simulink model "Suspension2_26_09_2023"  (R2022a)
settings: Solver=FixedStepAuto  StartTime=0.0  StopTime=10.0  FixedStep=0.001  RelTol=1e-3
undefined symbols (not defined in the file): a, alpha, area, b, beta, c, Force_rear_tyre, gamma, k, m, niu, theta1, theta2
libraries: simulink x1
settings Model: Creator=oltea  LastModifiedBy=oltea
settings DataIOCC: ReturnWorkspaceOutputs=off

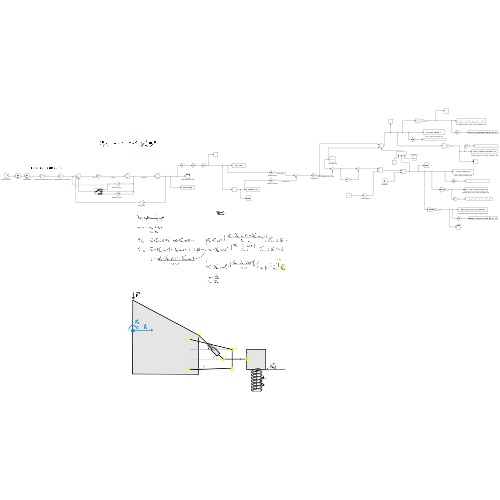
[thumbnail: Simulink's stored preview of the top-level diagram]
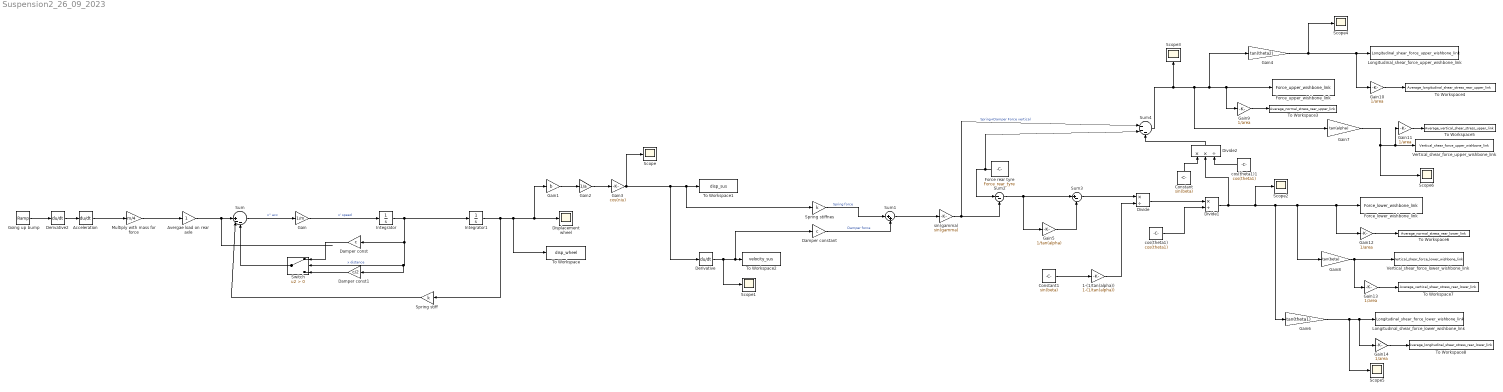
== system Suspension2_26_09_2023 ==
  " Avergae load on rear axle" : Gain
  1-(1/tan(alpha)) : Gain  Gain=1-(1/tan(alpha))
  Acceleration : Derivative
  Constant : Constant  Value=sin(beta)
  Constant1 : Constant  Value=sin(beta)
  Damper const : Gain  Gain=c
  Damper const1 : Gain  Gain=c/2
  Damper constant : Gain  Gain=c
  Derivative : Derivative
  Derivative2 : Derivative
  Displacement wheel : Scope
  Divide : Product  Inputs=*/
  Divide1 : Product  Inputs=*/
  Divide2 : Product  Inputs=**/
  Force rear tyre : Constant  Value=Force_rear_tyre
  Force_lower_wishbone_link : ToWorkspace  VariableName=Force_lower_wishbone_link  SampleTime=-1
  Force_upper_wishbone_link : ToWorkspace  VariableName=Force_upper_wishbone_link  SampleTime=-1
  Gain : Gain  Gain=1/m
  Gain1 : Gain  Gain=b
  Gain{9..14} (6 alike) : Gain  Gain=1/area
  Gain2 : Gain  Gain=1/a
  Gain3 : Gain  Gain=cos(niu)
  Gain4 : Gain  Gain=tan(theta2)
  Gain5 : Gain  Gain=1/tan(alpha)
  Gain6 : Gain  Gain=tan(theta1)
  Gain7 : Gain  Gain=tan(alpha)
  Gain8 : Gain  Gain=tan(beta)
  Going up bump : simulink/Sources/Ramp  slope=0.42  start=0  InitialOutput=7
  Integrator : Integrator
  Integrator1 : Integrator
  Longitudinal_shear_force_lower_wishbone_link : ToWorkspace  VariableName=Longitudinal_shear_force_lower_wishbone_link  SampleTime=-1
  Longitudinal_shear_force_upper_wishbone_link : ToWorkspace  VariableName=Longitudinal_shear_force_upper_wishbone_link  SampleTime=-1
  Multiply with mass for force : Gain  Gain=m/4
  Scope{,1..6} (7 alike) : Scope
  Spring stiff : Gain  Gain=k
  Spring stiffnes : Gain  Gain=k
  Sum : Sum  Inputs=||+--
  Sum1 : Sum  Inputs=|++
  Sum2 : Sum  Inputs=|--
  Sum3 : Sum  Inputs=|+-
  Sum4 : Sum  Inputs=|---
  Switch : Switch  Criteria=u2 > Threshold  SaturateOnIntegerOverflow=off  InputSameDT=off
  To Workspace : ToWorkspace  VariableName=disp_wheel  SampleTime=-1
  To Workspace1 : ToWorkspace  VariableName=disp_sus  SampleTime=-1
  To Workspace2 : ToWorkspace  VariableName=velocity_sus  SampleTime=-1
  To Workspace3 : ToWorkspace  VariableName=Average_normal_stress_rear_upper_link  SampleTime=-1
  To Workspace4 : ToWorkspace  VariableName=Average_longitudinal_shear_stress_rear_upper_link  SampleTime=-1
  To Workspace5 : ToWorkspace  VariableName=Average_vertical_shear_stress_upper_link  SampleTime=-1
  To Workspace6 : ToWorkspace  VariableName=Average_normal_stress_rear_lower_link  SampleTime=-1
  To Workspace7 : ToWorkspace  VariableName=Average_vertical_shear_stress_rear_lower_link  SampleTime=-1
  To Workspace8 : ToWorkspace  VariableName=Average_longitudinal_shear_stress_rear_lower_link  SampleTime=-1
  Vertical_shear_force_lower_wishbone_link : ToWorkspace  VariableName=Vertical_shear_force_lower_wishbone_link  SampleTime=-1
  Vertical_shear_force_upper_wishbone_link : ToWorkspace  VariableName=Vertical_shear_force_upper_wishbone_link  SampleTime=-1
  cos(theta1) : Constant  Value=cos(theta1)
  cos(theta1)1 : Constant  Value=cos(theta1)
  sin(gamma) : Gain  Gain=sin(gamma)
  wires:
  Switch/1 -> Sum/3
  Damper const1/1 -> Switch/3
  Spring stiff/1 -> Sum/2
  Integrator/1 -> Damper const1/1, Switch/2, Damper const/1, Integrator1/1  "x distance"
  Integrator1/1 -> Spring stiff/1, To Workspace/1, Gain1/1, Displacement wheel/1
  Damper const/1 -> Switch/1
  Sum/1 -> Gain/1  "x'' acc"
  Gain/1 -> Integrator/1  "x' speed"
  Going up bump/1 -> Derivative2/1
  Derivative2/1 -> Acceleration/1
  Acceleration/1 -> Multiply with mass for force/1
  Gain1/1 -> Gain2/1
  Gain2/1 -> Gain3/1
  Gain3/1 -> Scope/1, Derivative/1, Spring stiffnes/1, To Workspace1/1
  Derivative/1 -> Scope1/1, Damper constant/1, To Workspace2/1
  Spring stiffnes/1 -> Sum1/1  "Spring force"
  Damper constant/1 -> Sum1/2  "Damper force"
  Sum1/1 -> sin(gamma)/1
  Force rear tyre/1 -> Sum4/2, Sum2/1
  sin(gamma)/1 -> Sum4/1, Sum2/2  "Spring+Damper Force vertical"
  Sum2/1 -> Gain5/1, Sum3/1
  Gain5/1 -> Sum3/2
  Sum3/1 -> Divide/1
  1-(1/tan(alpha))/1 -> Divide/2
  Divide/1 -> Divide1/1
  cos(theta1)/1 -> Divide1/2
  Divide1/1 -> Scope2/1, Gain6/1, Gain8/1, Gain12/1, Force_lower_wishbone_link/1, Divide2/2
  Constant1/1 -> 1-(1/tan(alpha))/1
  Sum4/1 -> Gain7/1, Gain4/1, Gain9/1, Force_upper_wishbone_link/1, Scope3/1
  Constant/1 -> Divide2/1
  Divide2/1 -> Sum4/3
  cos(theta1)1/1 -> Divide2/3
  Gain4/1 -> Scope4/1, Gain10/1, Longitudinal_shear_force_upper_wishbone_link/1
  Gain6/1 -> Scope5/1, Gain14/1, Longitudinal_shear_force_lower_wishbone_link/1
  Gain7/1 -> Scope6/1, Gain11/1, Vertical_shear_force_upper_wishbone_link/1
  Gain8/1 -> Gain13/1, Vertical_shear_force_lower_wishbone_link/1
  Gain9/1 -> To Workspace3/1
  Gain10/1 -> To Workspace4/1
  Gain11/1 -> To Workspace5/1
  Gain12/1 -> To Workspace6/1
  Gain13/1 -> To Workspace7/1
  Gain14/1 -> To Workspace8/1
  Multiply with mass for force/1 -> " Avergae load on rear axle"/1
  " Avergae load on rear axle"/1 -> Sum/1
